simulink subsystem "servo_actuator"  (R2026a)
settings: Solver=VariableStepAuto
undefined symbols (not defined in the file): act_anglelimit, act_backlash, act_deadtime, act_freq, act_gear_ratio, act_ratelimit, canard_cant_zero, samplingtime_motor
libraries: simulink x1, aerolibactuator x1
settings Model: Creator=joedo  LastModifiedBy=trist

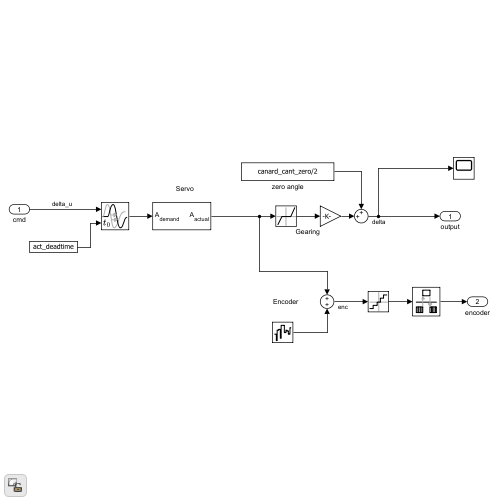
[thumbnail: Simulink's stored preview of the top-level diagram]
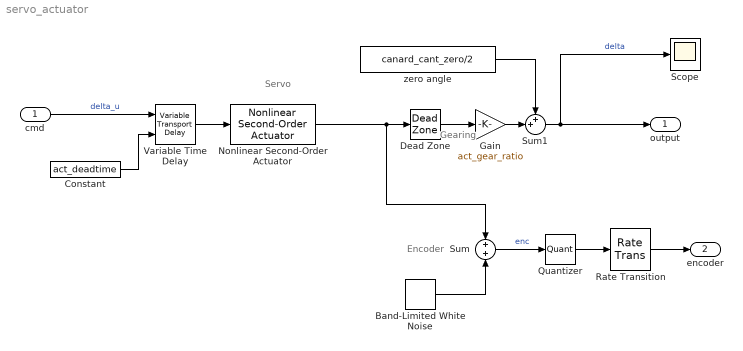
== system servo_actuator ==
  note: Servo
  note: Gearing
  note: Encoder
  cmd : Inport
  Band-Limited White Noise : simulink/Sources/Band-Limited White Noise  Cov=[1e-8]/2  Ts=samplingtime_motor  seed=[245637]
  Constant : Constant  Value=act_deadtime
  Dead Zone : DeadZone  LowerValue=-deg2rad(act_backlash)/2  UpperValue=deg2rad(act_backlash)/2
  Gain : Gain  Gain=act_gear_ratio
  Nonlinear Second-Order Actuator : aerolibactuator/Nonlinear Second-Order Actuator  wn_fin=act_freq/2  z_fin=act_damping  fin_max=deg2rad(act_anglelimit)  fin_min=-deg2rad(act_anglelimit)  fin_maxrate=deg2rad(act_ratelimit)/2  fin_act_0=0  fin_act_vel=0
  Quantizer : Quantizer  QuantizationInterval=deg2rad(0.1)
  Rate Transition : RateTransition  OutPortSampleTime=samplingtime_motor
  Scope : Scope
      settings: ActiveDisplayYMinimum=-0.080680107009746121  ActiveDisplayYMaximum=0.014674594481400401  DataLoggingVariableName=ScopeData4
  Sum : Sum
  Sum1 : Sum  Inputs=++|
  Variable Time Delay : VariableTransportDelay  PadeOrder=2
  zero angle : Constant  Value=canard_cant_zero/2
  output : Outport
  encoder : Outport  Port=2  PortDimensions=1
  wires:
  Sum1/1 -> output/1, Scope/1  "delta"
  cmd/1 -> Variable Time Delay/1  "delta_u"
  Band-Limited White Noise/1 -> Sum/2
  Variable Time Delay/1 -> Nonlinear Second-Order Actuator/1
  Constant/1 -> Variable Time Delay/2
  Nonlinear Second-Order Actuator/1 -> Dead Zone/1, Sum/1
  zero angle/1 -> Sum1/1
  Dead Zone/1 -> Gain/1
  Gain/1 -> Sum1/2
  Sum/1 -> Quantizer/1  "enc"
  Quantizer/1 -> Rate Transition/1
  Rate Transition/1 -> encoder/1
